simulink model "malha"  (Simulink 8.3)
settings: Solver=ode45  StartTime=0.0  StopTime=10.0  RelTol=1e-3
libraries: dspsrcs4 x1, simulink x1
settings Model: Creator=Jônatas  LastModifiedBy=Jônatas
settings DataIOCC: SignalLoggingSaveFormat=Dataset
settings DebuggingCC: UnderspecifiedInitializationDetection=Simplified  StateNameClashWarn=none
settings GRTTargetCC: CombineOutputUpdateFcns=on  GRTInterface=off
settings ConfigurationSet: Description=SimMechanics 2G

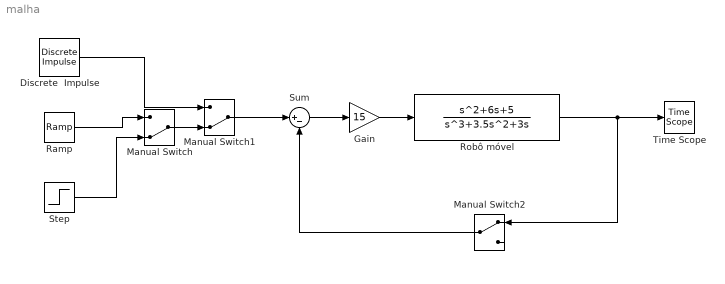
== system malha ==
  Discrete  Impulse : dspsrcs4/Discrete  Impulse  Delay=0  SampleTime=1  FrameSample=1  dataType=double  isSigned=on  wordLen=16  udDataType=sfix(16)  fracBitsMode=Best precision  numFracBits=15  OutDataTypeStr=double  LastOutDataTypeStr=double
  Gain : Gain  Gain=15
  Manual Switch : ManualSwitch  CurrentSetting=0
  Manual Switch1 : ManualSwitch  CurrentSetting=0
  Manual Switch2 : ManualSwitch
  Ramp : simulink/Sources/Ramp  slope=1  start=0  X0=0
  Robô móvel : TransferFcn  Numerator=[1 6 5]  Denominator=[1 3.5 3 0]
  Step : Step  SampleTime=0
  Sum : Sum  Inputs=|+-
  Time Scope : TimeScope  DefaultConfigurationName=spbscopes.TimeScopeBlockCfg  ScopeSpecification=DataTag0
  wires:
  Gain/1 -> Robô móvel/1
  Step/1 -> Manual Switch/2
  Ramp/1 -> Manual Switch/1
  Discrete  Impulse/1 -> Manual Switch1/1
  Manual Switch/1 -> Manual Switch1/2
  Sum/1 -> Gain/1
  Manual Switch1/1 -> Sum/1
  Robô móvel/1 -> Manual Switch2/1, Time Scope/1
  Manual Switch2/1 -> Sum/2
